simulink model "RadarLidarFusion"  (R2021b)
settings: Solver=FixedStepDiscrete  StartTime=0.1  StopTime=11.3  FixedStep=0.1  RelTol=1e-3
PreLoadFcn:
  | %Load the scnenario recording
  | load('RadarAndLidarTrackFusionScenario.mat')
  | 
  | rng(2019);
  | 
  | %RadarTrackBus
  | if ~exist('RadarTrackBus','var')
  |     % Sample Track
  |     sampleTrack =  struct('TrackID', uint32(1), ...
  |             'BranchID', uint32(1), ...
  |          'SourceIndex', uint32(1), ...
  |           'UpdateTime', double(zeros(1)), ...
  |                  'Age', uint32(1), ...
  |                'State', double(zeros(7,1)), ...
  |      'StateCovariance', double(zeros(7,7)), ...
  |      'StateParameters', struct(...
  |         'Frame',  fusionCoordinateFrameType.Rectangular,...
  |         'Position', double(zeros(1,3)), ...
  |         'Velocity', double(zeros(1,3))), ...
  |        'ObjectClassID', double(zeros(1)), ...
  |           'TrackLogic', trackLogicType(1), ...
  |      'TrackLogicState', false(1,10), ...
  |          'IsConfirmed', false, ...
  |            'IsCoasted', false, ...
  |       'IsSelfReported', false, ...
  |     'ObjectAttributes', struct('TargetIndex' , double(0)));
  | 
  |     %array of tracks
  |     tracks = repmat(sampleTrack,[100 1]);
  |     % Bus structure
  |     busFormat = struct('NumTracks',0,'Tracks',tracks);
  |     % Create Simulink.Bus
  |     busName = 'RadarTrackBus';
  |     theBus = Simulink.Bus.createObject(busFormat);
  |     tmpBusName = theBus.busName;
  |     evalin('base',[ busName ' = ' tmpBusName ';','clear ' tmpBusName]);
  | end
  | 
  | 
  | 
  | %Lidar Track Bus
  | if ~exist('LidarTrackBus','var')
  |     % Sample Track
  |     sampleTrack =  struct('TrackID', uint32(1), ...
  |             'BranchID', uint32(1), ...
  |          'SourceIndex', uint32(1), ...
  |           'UpdateTime', double(zeros(1)), ...
  |                  'Age', uint32(1), ...
  |                'State', double(zeros(10,1)), ...
  |      'StateCovariance', double(zeros(10,10)), ...
  |      'StateParameters', struct(...
  |         'Frame',  fusionCoordinateFrameType.Rectangular,...
  |         'Position', double(zeros(1,3)), ...
  |         'Velocity', double(zeros(1,3))), ...
  |        'ObjectClassID', double(zeros(1)), ...
  |           'TrackLogic', trackLogicType(1), ...
  |      'TrackLogicState', false(1,10), ...
  |          'IsConfirmed', false, ...
  |            'IsCoasted', false, ...
  |       'IsSelfReported', false, ...
  |     'ObjectAttributes', struct('TargetIndex' , double(0)));
  | 
  |     %array of tracks
  |     tracks = repmat(sampleTrack,[100 1]);
  |     % Bus structure
  |     busFormat = struct('NumTracks',0,'Tracks',tracks);
  |     % Create Simulink.Bus
  |     busName = 'LidarTrackBus';
  |     theBus = Simulink.Bus.createObject(busFormat);
  |     tmpBusName = theBus.busName;
  |     evalin('base',[ busName ' = ' tmpBusName ';','clear ' tmpBusName])
  | end
  | 
  | %lidar det bus
  | if ~exist('detectionBus','var')
  |     % Sample detection
  |     sampleDetection =struct('SensorIndex',1,...
  |                'Time',0,...
  |                'Measurement',zeros(7,1),...
  |                'MeasurementNoise',eye(7),...
  |                'ObjectClassID',0,...
  |                'MeasurementParameters',struct('OriginPosition',zeros(3,1),...
  |                'Frame',fusionCoordinateFrameType(1), ...
  |                'OriginVelocity',double(zeros(3,1)),...
  |                'Orientation',double(zeros(3,3))) ,...
  |                'ObjectAttributes',struct('TargetIndex',1));
  |     % Array of detections
  |     dets = repmat(sampleDetection,[100 1]);
  |     % Bus structure
  |     busFormat = struct('NumDetections',0,'Detections',dets);
  |     % Create Simulink.Bus
  |     busName = 'detectionBus';
  |     theBus = Simulink.Bus.createObject(busFormat);
  |     tmpBusName = theBus.busName;
  |     evalin('base',[ busName ' = ' tmpBusName ';','clear ' tmpBusName])
  | end
  | 
  | %Radar det bus
  | if ~exist('RadarDetBus','var')
  |     % Sample detection
  |     measPram=struct('Frame',fusionCoordinateFrameType(1),...
  |                 'OriginPosition',double(zeros(3,1)),...
  |                 'OriginVelocity',double(zeros(3,1)),...
  |                 'Orientation',double(zeros(3,3)),...
  |                 'HasElevation',false,...
  |                 'HasVelocity',false);
  |     sampleDetection =struct('Time',double(1),...
  |                 'Measurement',double(zeros(3,1)),...
  |                 'MeasurementNoise',double(zeros(3)),...
  |                 'SensorIndex',double(0),...
  |                 'ObjectClassID',double(0),...
  |                'MeasurementParameters',repmat(measPram,2,1) ,...
  |                'ObjectAttributes',struct('TargetIndex',0,'SNR',0));
  |     % Array of detections
  |     dets = repmat(sampleDetection,[200 1]);
  |     % Bus structure
  |     busFormat = struct('Detections',dets,'NumDetections',0);
  |     % Create Simulink.Bus
  |     busName = 'RadarDetBus';
  |     theBus = Simulink.Bus.createObject(busFormat);
  |     tmpBusName = theBus.busName;
  |     evalin('base',[ busName ' = ' tmpBusName ';','clear ' tmpBusName])
  | end
  | 
  | % Follow same steps as detectionBus for segmentationBus
  | if ~exist('segmentationBus','var')
  |     % Bus structure
  |     sampleSeg = struct('ObstacleIndices',false(57600,1),'GroundIndices',false(57600,1),'CroppedIndices',false(57600,1));
  |     segBus = Simulink.Bus.createObject(sampleSeg);
  | 
  |     % Clear original bus and create desired bus name
  |     segmentationBus = eval(segBus.busName);
  |     clear(segBus.busName);
  | end
  | 
  | %Radar sensor Config
  | radarSensorConfig = helperSensorConfigCell2struct();
  | %Fuser SourceConfig
  | SourceConfig = FuserSourceConfig();
  | %SensorResolution
  | load('radarSensorResolution.mat')
undefined symbols (not defined in the file or in its folder): fusionCoordinateFrameType, matlabshared
libraries: drivingscenarioandsensors x4, motalgorithmslib x3, trackingutilitieslib x2
CloseFcn:
  | % Close opened figure
  | fig = findall(0,'Tag','lidarRadarTrackFusionSimulinkExampleDisplay');
  | delete(fig);
settings Model: Creator=The MathWorks, Inc.  LastModifiedBy=ghisl

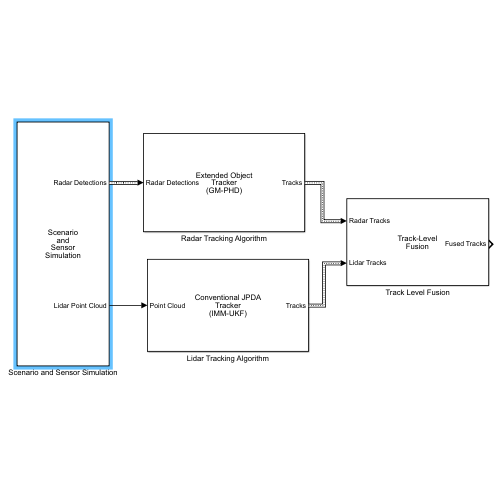
[thumbnail: Simulink's stored preview of the top-level diagram]
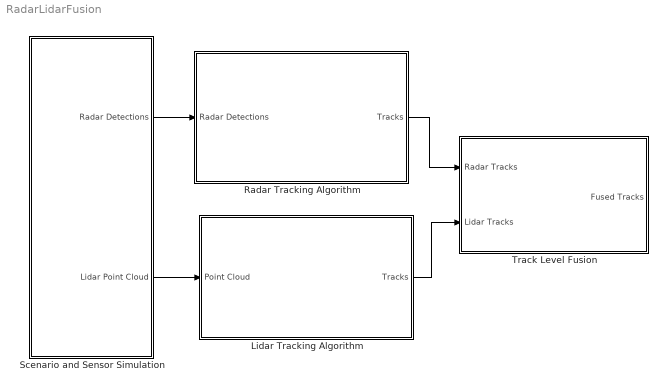
== system RadarLidarFusion ==
  Lidar Tracking Algorithm : Subsystem
      mask Display: disp('Conventional JPDA\nTracker\n(IMM-UKF)');
  Radar Tracking Algorithm : Subsystem
      mask Display: disp('Extended Object\nTracker\n(GM-PHD)')
  Scenario and Sensor Simulation : Subsystem
      mask Display: disp('Scenario\nand\nSensor\nSimulation');
  Track Level Fusion : Subsystem
      mask Display: disp('Track-Level\nFusion');
  wires:
  Lidar Tracking Algorithm/1(Tracks) -> Track Level Fusion/2(Lidar Tracks)
  Radar Tracking Algorithm/1(Tracks) -> Track Level Fusion/1(Radar Tracks)
  Scenario and Sensor Simulation/1(Radar Detections) -> Radar Tracking Algorithm/1(Radar Detections)
  Scenario and Sensor Simulation/2(Lidar Point Cloud) -> Lidar Tracking Algorithm/1(Point Cloud)

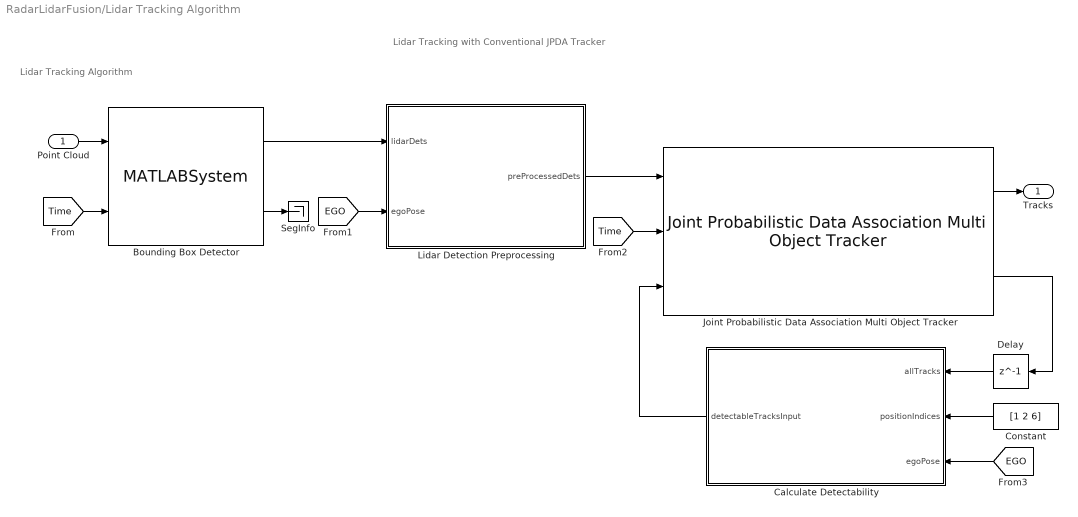
== system RadarLidarFusion/Lidar Tracking Algorithm ==
  note: Lidar Tracking Algorithm
  note: Lidar Tracking with Conventional JPDA Tracker
  Point Cloud : Inport
  Bounding Box Detector : MATLABSystem  System=HelperBoundingBoxDetectorBlk  DetectionBusName=detectionBus  SegmentationBusName=segmentationBus  NumLidarPoints=57600  XLimits=[ -120, 120 ]  YLimits=[ -20, 20 ]  ZLimits=[ -2, 5]  GroundMaxDistance=0.3  GroundReferenceVector=[ 0, 0, 1 ]  GroundMaxAngularDistance=5  SegmentationMinDistance=1.9  MinDetectionsPerCluster=2  MaxZDistanceCluster=3  MinZDistanceCluster=-3  EgoVehicleRadius=0.5  MeasurementNoise=blkdiag(0.05*eye(3),25,2*eye(3))  MeasurementParameters=struct('Frame',fusionCoordinateFrameType(1),'OriginPosition',zeros(3,1), 'OriginVelocity',zeros(3,1),'Orientation',eye(3))  SimulateUsing=Interpreted execution
      mask Type: HelperBoundingBoxDetectorBlk
      mask Display:
      | disp('Helper\nBounding\nBox\nDetector');
      | port_label('input',1,'Point Cloud');
      | port_label('input',2,'Time');
      | port_label('output',1,'Detections');
      | port_label('output',2,'SegmentationInfo');
  Calculate Detectability : MATLAB Function  TreatAsAtomicUnit=on
  Constant : Constant  Value=[1 2 6]
  Delay : Delay  DelayLength=1
  Joint Probabilistic Data Association Multi Object Tracker : motalgorithmslib/Joint Probabilistic Data Association Multi Object Tracker  TrackerIndex=uint32( 2 )  FilterInitializationFcn=helperInitIMMUKFFilter  MaxNumEvents=inf  EventGenerationFcn=jpdaEvents  MaxNumTracks=100  MaxNumSensors=20  TimeTolerance=1e-5  OOSMHandling=Terminate  StateParametersSimulink=struct('Frame',fusionCoordinateFrameType.Rectangular,'Position', double(zeros(1,3)),'Velocity', double(zeros(1,3)));  HasStateParametersInput=off  SimulateUsing=Interpreted execution  AssignmentThreshold=[250 inf]  InitializationThreshold=0  DetectionProbability=0.9  ClutterDensity=1e-9  TrackLogic=History  pHistoryConfThreshold=[ 7, 10]  pHistoryDelThreshold=[ 8, 10 ]  pIntegratedConfThreshold=0.95  pIntegratedDelThreshold=0.1  HitMissThreshold=0.1  NewTargetDensity=1e-5  DeathRate=0.01  TimeInputSource=Input port  HasCostMatrixInput=off  HasDetectableTrackIDsInput=on  TentativeTracksOutputPort=off  AllTracksOutputPort=on  InfoOutputPort=off  BusNameSource=Auto  BusName=BusTrackerJPDA  BusName2Source=Auto  BusName2=BusTrackerInfo
      settings: SourceProductBaseCode=TF
  Lidar Detection Preprocessing : MATLAB Function  TreatAsAtomicUnit=on
  SegInfo : Terminator
  Tracks : Outport
  wires:
  Calculate Detectability/1(detectableTracksInput) -> Joint Probabilistic Data Association Multi Object Tracker/3
  Point Cloud/1 -> Bounding Box Detector/1
  Delay/1 -> Calculate Detectability/1(allTracks)
  Constant/1 -> Calculate Detectability/2(positionIndices)
  Joint Probabilistic Data Association Multi Object Tracker/1 -> Tracks/1
  Joint Probabilistic Data Association Multi Object Tracker/2 -> Delay/1
  Lidar Detection Preprocessing/1(preProcessedDets) -> Joint Probabilistic Data Association Multi Object Tracker/1
  Bounding Box Detector/1 -> Lidar Detection Preprocessing/1(lidarDets)
  [Time] -> Bounding Box Detector/2
  [EGO] -> Lidar Detection Preprocessing/2(egoPose)
  [Time] -> Joint Probabilistic Data Association Multi Object Tracker/2
  [EGO] -> Calculate Detectability/3(egoPose)
  Bounding Box Detector/2 -> SegInfo/1

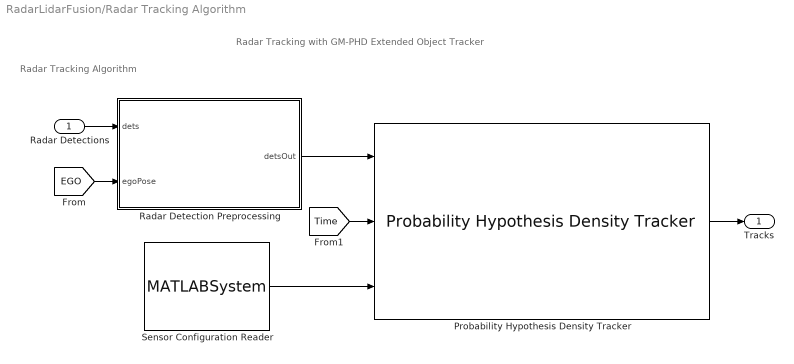
== system RadarLidarFusion/Radar Tracking Algorithm ==
  note: Radar Tracking Algorithm
  note: Radar Tracking with GM-PHD Extended Object Tracker
  Radar Detections : Inport
  Probability Hypothesis Density Tracker : motalgorithmslib/Probability Hypothesis Density Tracker  TrackerIndexSimulink=1  PartitioningFcn=helperDetectionPartitionFcn  AssignmentThreshold=320  MaxNumSensors=20  MaxNumTracks=100  SensorConfigurationExpression=radarSensorConfig  IsSensorConfigurationsInput=on  StateParametersSimulink="struct('Frame',  fusionCoordinateFrameType.Rectangular, 'Position', double(zeros(1,3)), 'Velocity', double(zeros(1,3)));"  IsStateParametersInput=off  SimulateUsing=Interpreted execution  BirthRate=1e-3  DeathRate=1e-6  ExtractionThreshold=0.85  ConfirmationThreshold=0.98  DeletionThreshold=1e-3  MergingThreshold=50  LabelingThresholds=[ 1.1, 1.01, 0 ]  TimeInputSource=Input port  TentativeTracksOutputPort=off  AllTracksOutputPort=off  InfoOutputPort=off  BusNameSource=Auto  BusName=BusTrackerPHD  BusName2Source=Auto  BusName2=BusTrackerPHDInfo
      settings: SourceProductBaseCode=TF
  Radar Detection Preprocessing : MATLAB Function  TreatAsAtomicUnit=on
  Sensor Configuration Reader : MATLABSystem  System=HelperSourceConfigReader  DataFile={ 'SensorConfigurations' }  BusNameSource=Auto  BusName=BusDataLog
      mask Type: HelperSourceConfigReader
      mask Display:
      | disp(['Helper' char(10) 'Sensor' char(10) 'Configurations' char(10) 'Reader']);
      | port_label('output',1,['Sensor' char(10) 'Conf']);
  Tracks : Outport
  wires:
  Radar Detections/1 -> Radar Detection Preprocessing/1(dets)
  Radar Detection Preprocessing/1(detsOut) -> Probability Hypothesis Density Tracker/1
  Probability Hypothesis Density Tracker/1 -> Tracks/1
  Sensor Configuration Reader/1 -> Probability Hypothesis Density Tracker/3
  [EGO] -> Radar Detection Preprocessing/2(egoPose)
  [Time] -> Probability Hypothesis Density Tracker/2

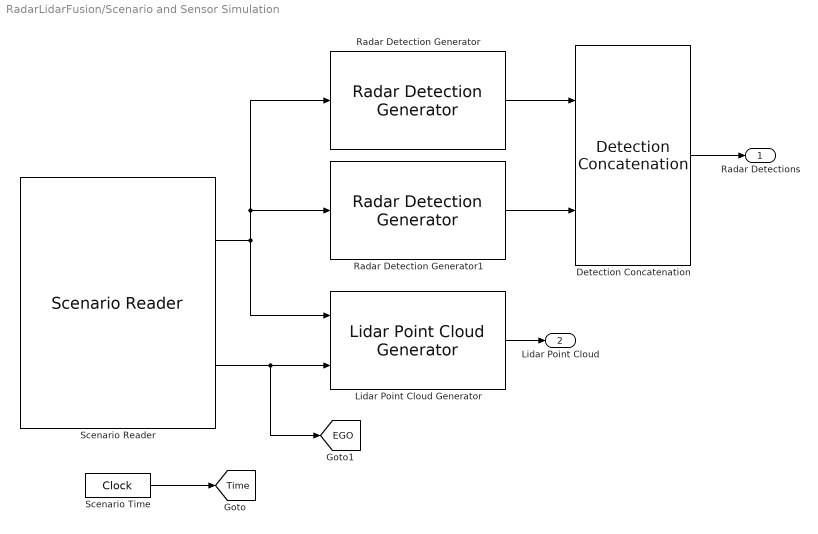
== system RadarLidarFusion/Scenario and Sensor Simulation ==
  Detection Concatenation : trackingutilitieslib/Detection Concatenation  NumInputs=2  BusNameSource=Auto  BusName=BusDetectionConcatenation  SimulateUsing=Interpreted execution
      settings: SourceProductBaseCode=AE,DR,TF,RA,UV,VE
  Lidar Point Cloud Generator : drivingscenarioandsensors/Lidar Point Cloud Generator  SensorIndex=5  UpdateInterval=0.1  SensorLocation=[0 0]  Height=2  Yaw=0  Pitch=0  Roll=0  DetectionCoordinates=Ego Cartesian  HasEgoVehicle=off  EgoVehicleActorID=1  HasRoadsInputPort=on  ActorProfilesSource=From Scenario Reader block  ActorProfilesVariableName=actor_profiles  MaxRange=120  RangeAccuracy=0.002  AzimuthResolution=0.2  ElevationResolution=1.25  AzimuthLimits=[ -180, 180 ]  ElevationLimits=[ -30, 10 ]  HasNoise=on
      settings: SourceProductBaseCode=DR
  Radar Detection Generator : drivingscenarioandsensors/Radar Detection Generator  SensorIndex=1  UpdateInterval=0.1  SensorLocation=[ 3.7, 0 ]  Height=0.6  Yaw=0  Pitch=0  Roll=0  BusNameSource=Auto  BusName=BusRadarDetectionGenerator  MaxNumDetectionsSource=Property  MaxNumDetections=50  DetectionCoordinates=Sensor spherical  SimulateUsing=Interpreted execution  AzimuthResolution=6  ElevationResolution=10  RangeResolution=2.5  RangeRateResolution=1  AzimuthBiasFraction=0.1  ElevationBiasFraction=0.1  RangeBiasFraction=0.05  RangeRateBiasFraction=0.05  FieldOfView=[ 45, 5 ]  MaxRange=80  RangeRateLimits=[ -100, 100 ]  DetectionProbability=0.9  FalseAlarmRate=1e-6  ReferenceRange=100  ReferenceRCS=0  HasElevation=off  HasRangeRate=on  HasNoise=on  HasFalseAlarms=on  HasOcclusion=off  InitialSeedSource=Repeatable  InitialSeed=0  UsedSeed=matlabshared.tracking.internal.SimulinkUtilities.seedManager(gcb)  ActorProfilesSource=From Scenario Reader block  ActorProfilesParameters=driving.internal.ActorProfilesRadarParameters  ActorProfilesExpression=struct( 'ClassID', 0, 'Length', 4.7, 'Width', 1.8, 'Height', 1.4, 'OriginOffset', [ -1.35, 0, 0 ], 'RCSPattern', [ 10, 10; 10, 10 ], 'RCSAzimuthAngles', [ -180, 180 ], 'RCSElevationAngles', [ -90, 90 ] )
      settings: SourceProductBaseCode=DR
  Radar Detection Generator1 : drivingscenarioandsensors/Radar Detection Generator  SensorIndex=2  UpdateInterval=0.1  SensorLocation=[ -1, 0 ]  Height=0.6  Yaw=180  Pitch=0  Roll=0  BusNameSource=Auto  BusName=BusRadarDetectionGenerator  MaxNumDetectionsSource=Property  MaxNumDetections=50  DetectionCoordinates=Sensor spherical  SimulateUsing=Interpreted execution  AzimuthResolution=6  ElevationResolution=10  RangeResolution=2.5  RangeRateResolution=1  AzimuthBiasFraction=0.1  ElevationBiasFraction=0.1  RangeBiasFraction=0.05  RangeRateBiasFraction=0.05  FieldOfView=[ 45, 5 ]  MaxRange=80  RangeRateLimits=[ -100, 100 ]  DetectionProbability=0.9  FalseAlarmRate=1e-6  ReferenceRange=100  ReferenceRCS=0  HasElevation=off  HasRangeRate=on  HasNoise=on  HasFalseAlarms=on  HasOcclusion=off  InitialSeedSource=Repeatable  InitialSeed=0  UsedSeed=matlabshared.tracking.internal.SimulinkUtilities.seedManager(gcb)  ActorProfilesSource=From Scenario Reader block  ActorProfilesParameters=driving.internal.ActorProfilesRadarParameters  ActorProfilesExpression=struct( 'ClassID', 0, 'Length', 4.7, 'Width', 1.8, 'Height', 1.4, 'OriginOffset', [ -1.35, 0, 0 ], 'RCSPattern', [ 10, 10; 10, 10 ], 'RCSAzimuthAngles', [ -180, 180 ], 'RCSElevationAngles', [ -90, 90 ] )
      settings: SourceProductBaseCode=DR
  Scenario Reader : drivingscenarioandsensors/Scenario Reader  ScenarioSource=From workspace  ScenarioFileName=EgoVehicleGoesStraight.mat  ScenarioVariableName=RadarAndLidarTrackFusionScenario  OutputCoordinateSystem=Vehicle coordinates  EgoVehicleSource=Scenario  EgoVehicleActorID=1  OrientVehiclesOnRoad=off  OutputEgoVehiclePose=on  OutputEgoVehicleState=off  SampleTime=0.1  LaneBoundaryOutput=None  LaneBoundaryDistance=0:0.5:9.5  LaneBoundaryLocation=Center of lane markings  BusNameSource=Auto  BusName=BusActors  BusNumActorsSource=Scenario  BusNumActors=100  BusName2Source=Auto  BusName2=BusLaneBoundaries  BusNumLaneBoundariesSource=Scenario  BusNumLaneBoundaries=10  BusName3Source=Auto  BusName3=BusEgoActor  BusName4Source=Auto  BusName4=BusEgoState  ShowCoordinateLabels=on  SimulateUsing=Interpreted execution
  Scenario Time : DigitalClock  SampleTime=0.1
  Radar Detections : Outport
  Lidar Point Cloud : Outport  Port=2
  tag scope: EGO=global, Time=global
  wires:
  Scenario Reader/1 -> Radar Detection Generator/1, Radar Detection Generator1/1, Lidar Point Cloud Generator/1
  Scenario Time/1 -> [Time]
  Lidar Point Cloud Generator/1 -> Lidar Point Cloud/1
  Detection Concatenation/1 -> Radar Detections/1
  Scenario Reader/2 -> [EGO], Lidar Point Cloud Generator/2
  Radar Detection Generator/1 -> Detection Concatenation/1
  Radar Detection Generator1/1 -> Detection Concatenation/2

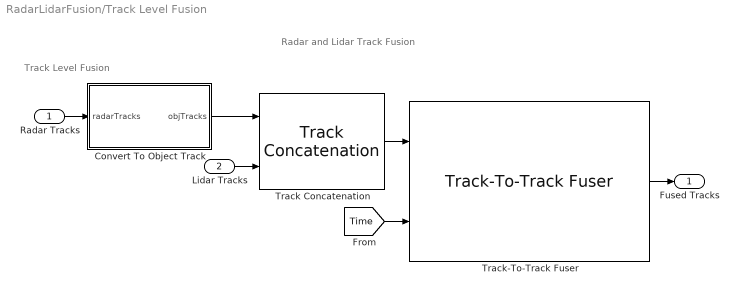
== system RadarLidarFusion/Track Level Fusion ==
  note: Track Level Fusion
  note: Radar and Lidar Track Fusion
  Radar Tracks : Inport
  Lidar Tracks : Inport  Port=2
  Convert To Object Track : MATLAB Function  TreatAsAtomicUnit=on
  Track Concatenation : trackingutilitieslib/Track Concatenation  NumInputs=2  BusNameSource=Auto  BusName=BusTrackConcatenation  SimulateUsing=Interpreted execution
      settings: SourceProductBaseCode=AE,DR,TF,RA,UV,VE
  Track-To-Track Fuser : motalgorithmslib/Track-To-Track Fuser  FuserIndex=1  Assignment=MatchPairs  AssignmentThreshold=[250 inf]  MaxNumCentralTracks=100  MaxNumSources=20  SourceConfigurationExpression=SourceConfig  IsSourceConfigurationsInput=off  StateParametersSimulink=struct  IsStateParametersInput=off  SimulateUsing=Interpreted execution  ConfirmationThreshold=[3 5]  DeletionThreshold=[ 5, 5 ]  CentralTrackStateSize=10  CentralObjectAttributes=repmat(struct('TargetIndex' , double(0)),20,1);  StateTransitionFcn=helperctcuboid  ProcessNoise=diag([1 3 1])  HasAdditiveProcessNoise=off  StateFusion=Custom  CustomStateFusionFcn=helperRadarLidarFusionFunction  StateFusionParamSource=Auto  StateFusionCross=0.4  StateFusionIntersection=det  FuseConfirmedOnly=on  FuseCoasted=off  TimeInputSource=Input port  TentativeTracksOutputPort=off  AllTracksOutputPort=off  InfoOutputPort=off  BusNameSource=Auto  BusName=BusTrackFuser  BusName2Source=Auto  BusName2=BusTrackFuserInfo
      settings: SourceProductBaseCode=TF
  Fused Tracks : Outport
  wires:
  Track Concatenation/1 -> Track-To-Track Fuser/1
  Convert To Object Track/1(objTracks) -> Track Concatenation/1
  Lidar Tracks/1 -> Track Concatenation/2
  Track-To-Track Fuser/1 -> Fused Tracks/1
  Radar Tracks/1 -> Convert To Object Track/1(radarTracks)
  [Time] -> Track-To-Track Fuser/2

== matlab function RadarLidarFusion/Track Level Fusion/Convert To Object Track ==
  data: radarTracks input size=[1,1]; objTracks output Bus: RadarTrackBus size=[1,1]

function objTracks = toObjectTrack(radarTracks)
% This function adds 'BranchID' field to the output bus which is expected by the Track
% Concatenation block but is not available in trackerPHD output.

trk  = struct('TrackID', uint32(1), ...
            'BranchID', uint32(1), ...
         'SourceIndex', uint32(1), ...
          'UpdateTime', double(zeros(1)), ...
                 'Age', uint32(1), ...
               'State', double(zeros(7,1)), ...
     'StateCovariance', double(zeros(7,7)), ...
     'StateParameters', struct(...
        'Frame',  fusionCoordinateFrameType.Rectangular,...
        'Position', double(zeros(1,3)), ...
        'Velocity', double(zeros(1,3))), ...
       'ObjectClassID', double(zeros(1)), ...
          'TrackLogic', trackLogicType(1), ...
     'TrackLogicState', false(1,10), ...
         'IsConfirmed', false, ...
           'IsCoasted', false, ...
      'IsSelfReported', false, ...
    'ObjectAttributes', struct('TargetIndex' , double(0)));


objTracks = struct('NumTracks',radarTracks.NumTracks,'Tracks',repmat(trk, 100,1));

for i = 1 : radarTracks.NumTracks
    tr = radarTracks.Tracks(i);
    
    objTracks.Tracks(i).TrackID = tr.TrackID;        
    objTracks.Tracks(i).SourceIndex= tr.SourceIndex;
    objTracks.Tracks(i).UpdateTime= tr.UpdateTime;
    objTracks.Tracks(i).Age= uint32(tr.Age);
    objTracks.Tracks(i).ObjectClassID= tr.ObjectClassID;
    objTracks.Tracks(i).IsConfirmed= tr.IsConfirmed;
    objTracks.Tracks(i).IsCoasted= tr.IsCoasted;
    objTracks.Tracks(i).IsSelfReported= tr.IsSelfReported;
    objTracks.Tracks(i).State=tr.State ;
    objTracks.Tracks(i).StateCovariance=tr.StateCovariance;
end


end

== matlab function RadarLidarFusion/Lidar Tracking Algorithm/Calculate Detectability ==
  settings: updateMethod=DISCRETE  sampleTime=0.1
  data allTracks settings: description=All Tracks
  data: allTracks input; detectableTracksInput output size=[100 2]; positionIndices input size=[1 3]; egoPose input size=[1 1]
function detectableTracksInput = CalculateDetectability(allTracks, positionIndices,egoPose)
% This function calculates the probability of detection for each track. The
% helperCalcDetectability function is used to compute the probability after
% extracting the tracks from the bus.

egoMeasParams = struct('Frame',fusionCoordinateFrameType(1),...
    'OriginPosition',egoPose.Position(:),...
    'OriginVelocity',egoPose.Velocity(:),...
    'Orientation', rotmat(quaternion([egoPose.Yaw, egoPose.Pitch egoPose.Roll],'eulerd','ZYX','frame'),'frame')...
    );

tracks = allTracks.Tracks(1:allTracks.NumTracks);
detectableTracksInput = helperCalculateDetectability(tracks, positionIndices,egoMeasParams);
end

== matlab function RadarLidarFusion/Lidar Tracking Algorithm/Lidar Detection Preprocessing ==
  data: preProcessedDets output Bus: detectionBus size=[1,1]; lidarDets input Bus: detectionBus size=[1,1]; egoPose input size=[1 1]
function preProcessedDets = preProcessDetections(lidarDets, egoPose)
% Add Ego-Vehicle's information to the detection's MeasurementParameters to
% track state in the scenario frame.

preProcessedDets = lidarDets;
egoMeasParams = struct('Frame',fusionCoordinateFrameType(1),...
    'OriginPosition',egoPose.Position(:),...
    'OriginVelocity',egoPose.Velocity(:),...
    'Orientation', rotmat(quaternion([egoPose.Yaw, egoPose.Pitch egoPose.Roll],'eulerd','ZYX','frame'),'frame')...
    );
for i = 1:lidarDets.NumDetections
    preProcessedDets.Detections(i).MeasurementParameters.Frame = egoMeasParams.Frame;
    preProcessedDets.Detections(i).MeasurementParameters.OriginPosition = egoMeasParams.OriginPosition;
    preProcessedDets.Detections(i).MeasurementParameters.OriginVelocity = egoMeasParams.OriginVelocity;
    preProcessedDets.Detections(i).MeasurementParameters.Orientation = egoMeasParams.Orientation;

end
end

== matlab function RadarLidarFusion/Radar Tracking Algorithm/Radar Detection Preprocessing ==
  data: dets input; detsOut output Bus: RadarDetBus; egoPose input; radarSensorResolution parameter
function detsOut = preprocessDetections(dets,egoPose,radarSensorResolution)
% Detections cannot report an uncertainty better than sensor's resolution
% and must be updated to include ego vehicle or INS information

% Update Measurement paramters
n = dets.NumDetections;
% Sample detection
measPram=struct('Frame',fusionCoordinateFrameType(1),...
    'OriginPosition',double(zeros(3,1)),...
    'OriginVelocity',double(zeros(3,1)),...
    'Orientation',double(zeros(3,3)),...
    'HasElevation',false,...
    'HasVelocity',false);
sampleDetection =struct('Time',double(1),...
    'Measurement',double(zeros(3,1)),...
    'MeasurementNoise',double(zeros(3)),...
    'SensorIndex',double(0),...
    'ObjectClassID',double(0),...
    'MeasurementParameters',repmat(measPram,2,1) ,...
    'ObjectAttributes',struct('TargetIndex',0,'SNR',0));
% Array of detections
sampleDets = repmat(sampleDetection,[200 1]);
detsOut = struct('Detections',sampleDets,'NumDetections',n);



for i = 1:n
    idx = dets.Detections(i).SensorIndex;
    res = radarSensorResolution(idx).SensorResolution;
    resNoise = diag(res.^2/4);
    
    detsOut.Detections(i).Time = dets.Detections(i).Time;
    detsOut.Detections(i).Measurement=  dets.Detections(i).Measurement;
    detsOut.Detections(i).MeasurementNoise=  dets.Detections(i).MeasurementNoise;
    detsOut.Detections(i).SensorIndex=  dets.Detections(i).SensorIndex;
    detsOut.Detections(i).ObjectClassID=  dets.Detections(i).ObjectClassID;
    detsOut.Detections(i).ObjectAttributes=  dets.Detections(i).ObjectAttributes;
    
    detsOut.Detections(i).MeasurementParameters(1).Frame(:) = fusionCoordinateFrameType(2);
    detsOut.Detections(i).MeasurementParameters(1).OriginPosition =dets.Detections(i).MeasurementParameters(1).OriginPosition;
    detsOut.Detections(i).MeasurementParameters(1).Orientation=dets.Detections(i).MeasurementParameters(1).Orientation;
    detsOut.Detections(i).MeasurementParameters(1).HasElevation=dets.Detections(i).MeasurementParameters(1).HasElevation;
    detsOut.Detections(i).MeasurementParameters(1).HasVelocity= dets.Detections(i).MeasurementParameters(1).HasVelocity;
    
    detsOut.Detections(i).MeasurementParameters(2).Frame(:) = fusionCoordinateFrameType(1);
    detsOut.Detections(i).MeasurementParameters(2).OriginPosition = egoPose.Position(:);
    detsOut.Detections(i).MeasurementParameters(2).OriginVelocity = egoPose.Velocity(:);
    detsOut.Detections(i).MeasurementParameters(2).Orientation = rotmat(quaternion([egoPose.Yaw egoPose.Pitch egoPose.Roll],'eulerd','ZYX','frame'),'frame')';
    detsOut.Detections(i).MeasurementNoise(1:2,1:2) = resNoise;
    detsOut.Detections(i).MeasurementNoise(3,3) = 0.5^2/4;
end

end
